simulink model "RLCpart2actual"  (R2018a)
settings: Solver=VariableStepAuto  StartTime=0.0  StopTime=2.0  RelTol=1e-3
settings Model: Creator=praty  LastModifiedBy=praty
settings DebuggingCC: LibraryContextMissingDiagnostic=warning
settings SFSimCC: SimUseLocalCustomCode=on
settings RTWCC: RTWUseLocalCustomCode=on

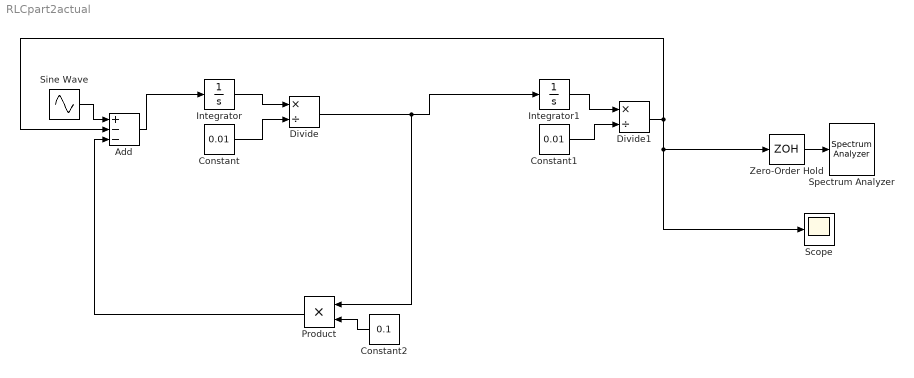
== system RLCpart2actual ==
  Add : Sum  Inputs=+--
  Constant : Constant  Value=0.01
  Constant1 : Constant  Value=0.01
  Constant2 : Constant  Value=0.1
  Divide : Product  Inputs=*/
  Divide1 : Product  Inputs=*/
  Integrator : Integrator
  Integrator1 : Integrator
  Product : Product
  Scope : Scope
  Sine Wave : Sin  SampleTime=0
  Spectrum Analyzer : SpectrumAnalyzer
  Zero-Order Hold : ZeroOrderHold  SampleTime=2^(-10)
  wires:
  Zero-Order Hold/1 -> Spectrum Analyzer/1
  Integrator/1 -> Divide/1
  Constant/1 -> Divide/2
  Integrator1/1 -> Divide1/1
  Constant1/1 -> Divide1/2
  Divide/1 -> Product/1, Integrator1/1
  Constant2/1 -> Product/2
  Add/1 -> Integrator/1
  Divide1/1 -> Scope/1, Zero-Order Hold/1, Add/2
  Product/1 -> Add/3
  Sine Wave/1 -> Add/1
